simulink model "controller"  (Simulink 4.00)
settings: Solver=ode45  StartTime=0.0  StopTime=10.0  RelTol=1e-3
settings Model: Creator=dan  LastModifiedBy=anton  ExtModeAutoUpdateStatusClock=off  BlockReductionOpt=off

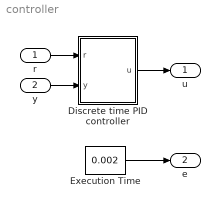
== system controller ==
  r : Inport  Port=1  LatchInput=off
  y : Inport  Port=2  LatchInput=off
  Discrete time PID controller : Subsystem  mask{K=0.96, Ti=0.12, Td=0.049, beta=0.5, N=10, h=0.006}
      settings: RTWFcnNameOpts=Auto  RTWFileNameOpts=Auto
  Execution Time : Constant  Value=0.002
  u : Outport  Port=1
  e : Outport  Port=2
  wires:
  Discrete time PID controller/1(u) -> u/1
  y/1 -> Discrete time PID controller/2(y)
  r/1 -> Discrete time PID controller/1(r)
  Execution Time/1 -> e/1

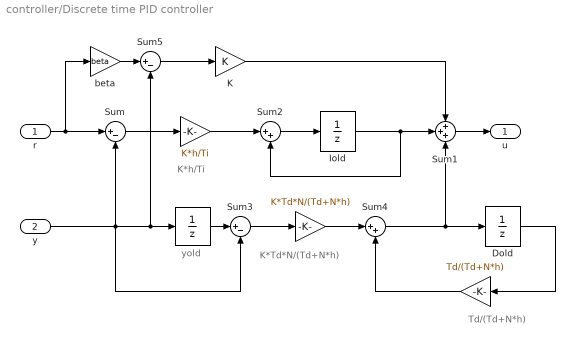
== system controller/Discrete time PID controller ==
  note: K*h/Ti
  note: K*Td*N/(Td+N*h)
  note: Td/(Td+N*h)
  note: yold
  r : Inport  Port=1  LatchInput=off
  y : Inport  Port=2  LatchInput=off
  " " : UnitDelay  X0=0  SampleTime=1
      settings: RTWStateStorageClass=Auto
  "   " : Gain  Gain=K*h/Ti  Multiplication=Element-wise(K.*u)  SaturateOnIntegerOverflow=on
  "             " : Gain  Gain=K*Td*N/(Td+N*h)  Multiplication=Element-wise(K.*u)  SaturateOnIntegerOverflow=on
  "              " : Gain  Orientation=left  Gain=Td/(Td+N*h)  Multiplication=Element-wise(K.*u)  SaturateOnIntegerOverflow=on
  Dold : UnitDelay  X0=0  SampleTime=1
      settings: RTWStateStorageClass=Auto
  "Iold " : UnitDelay  X0=0  SampleTime=1
      settings: RTWStateStorageClass=Auto
  K : Gain  Gain=K  Multiplication=Element-wise(K.*u)  SaturateOnIntegerOverflow=on
  Sum : Sum  Inputs=|+-  SaturateOnIntegerOverflow=on
  Sum1 : Sum  Inputs=+++  SaturateOnIntegerOverflow=on
  Sum2 : Sum  Inputs=|++  SaturateOnIntegerOverflow=on
  Sum3 : Sum  Inputs=|+-  SaturateOnIntegerOverflow=on
  Sum4 : Sum  Inputs=|++  SaturateOnIntegerOverflow=on
  Sum5 : Sum  Inputs=|+-  SaturateOnIntegerOverflow=on
  beta : Gain  Gain=beta  Multiplication=Element-wise(K.*u)  SaturateOnIntegerOverflow=on
  u : Outport  Port=1
  wires:
  y/1 -> Sum/2, Sum3/2, " "/1, Sum5/2
  r/1 -> Sum/1, beta/1
  Sum1/1 -> u/1
  K/1 -> Sum1/1
  Sum2/1 -> "Iold "/1
  Dold/1 -> "              "/1
  "             "/1 -> Sum4/1
  Sum3/1 -> "             "/1
  Sum4/1 -> Dold/1, Sum1/3
  " "/1 -> Sum3/1
  "Iold "/1 -> Sum2/2, Sum1/2
  "   "/1 -> Sum2/1
  Sum/1 -> "   "/1
  "              "/1 -> Sum4/2
  beta/1 -> Sum5/1
  Sum5/1 -> K/1
